simulink model "SMC"  (R2020b)
settings: Solver=VariableStepAuto  StartTime=0.0  StopTime=100  RelTol=1e-3
settings Model: Creator=Lenovo  LastModifiedBy=Lenovo
settings DataIOCC: ReturnWorkspaceOutputs=off
settings DebuggingCC: ArithmeticOperatorsInVariantConditions=warning
settings SFSimCC: SimUseLocalCustomCode=off  CustomCodeUndefinedFunction=UseInterfaceOnly
settings RTWCC: RTWUseLocalCustomCode=off

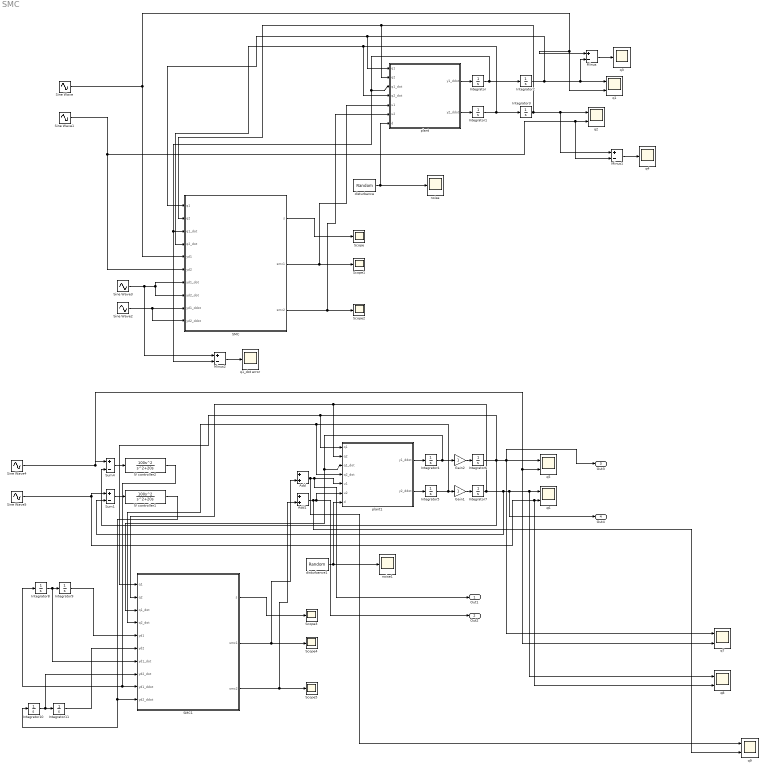
== system SMC ==
  Add : Sum
  Add1 : Sum
  Gain1 : Gain
  Gain2 : Gain
  IV controller1 : TransferFcn  Numerator=[100 0 0]  Denominator=[1 20 0]
  IV controller2 : TransferFcn  Numerator=[100 0 0]  Denominator=[1 20 0]
  Integrator{,1..11} (12 alike) : Integrator
  Minus : Sum  Inputs=+-
  Minus1 : Sum  Inputs=+-
  Minus2 : Sum  Inputs=+-
  SMC : MATLAB Function  TreatAsAtomicUnit=on
  SMC1 : MATLAB Function  TreatAsAtomicUnit=on
  Scope{,1..5} (6 alike) : Scope
  Sine Wave : Sin  Frequency=6  SampleTime=0.001
  Sine Wave1 : Sin  Frequency=6  SampleTime=0.001
  Sine Wave2 : Sin  Amplitude=-36  Frequency=6  SampleTime=0.001
  Sine Wave3 : Sin  Amplitude=6  Frequency=6  Phase=1.57  SampleTime=0.001
  Sine Wave4 : Sin  SampleTime=0.001
  Sine Wave5 : Sin  SampleTime=0.001
  Sum1 : Sum  Inputs=|+-
  Sum4 : Sum  Inputs=|+-
  disturbance : UniformRandomNumber  Minimum=0  Maximum=10  SampleTime=0.01
  disturbance1 : UniformRandomNumber  Minimum=-10  Maximum=10  SampleTime=0.001
  noise : Scope
  noise1 : Scope
  plant : MATLAB Function  TreatAsAtomicUnit=on
  plant1 : MATLAB Function  TreatAsAtomicUnit=on
  q{1..2,5..9} (7 alike) : Scope  NumInputPorts=2
  q1_dot error : Scope
  q3 : Scope
  q4 : Scope
  Out1 : Outport  VectorParamsAs1DForOutWhenUnconnected=off
  Out2 : Outport  Port=2  VectorParamsAs1DForOutWhenUnconnected=off
  Out3 : Outport  Port=3  VectorParamsAs1DForOutWhenUnconnected=off
  Out4 : Outport  Port=4  VectorParamsAs1DForOutWhenUnconnected=off
  wires:
  disturbance/1 -> plant/7(d), noise/1
  plant/2(y2_ddot) -> Integrator1/1
  SMC/1(s) -> Scope/1
  SMC/3(smc2) -> plant/6(u2), Scope2/1
  SMC/2(smc1) -> plant/5(u1), Scope1/1
  Integrator1/1 -> Integrator3/1, SMC/4(q2_dot), plant/4(q2_dot)
  plant/1(y1_ddot) -> Integrator/1
  Integrator2/1 -> Minus/2, q1/1, SMC/1(q1), plant/1(q1)
  Sine Wave/1 -> SMC/5(yd1), Minus/1, q1/2
  Sine Wave2/1 -> SMC/10(yd2_ddot), SMC/9(yd1_ddot)
  Minus/1 -> q3/1
  Sine Wave1/1 -> Minus1/2, q2/2, SMC/6(yd2)
  Integrator3/1 -> Minus1/1, q2/1, SMC/2(q2), plant/2(q2)
  Minus1/1 -> q4/1
  Integrator/1 -> Integrator2/1, Minus2/2, SMC/3(q1_dot), plant/3(q1_dot)
  Sine Wave3/1 -> Minus2/1, SMC/8(yd2_dot), SMC/7(yd1_dot)
  Minus2/1 -> q1_dot error/1
  Integrator11/1 -> SMC1/6(yd2)
  Sum1/1 -> IV controller1/1
  disturbance1/1 -> plant1/7(d), noise1/1
  Sine Wave5/1 -> q8/2, q6/2, Sum1/1
  Add1/1 -> q9/2, Out2/1, plant1/6(u2)
  Add/1 -> q9/1, Out1/1, plant1/5(u1)
  Integrator9/1 -> SMC1/5(yd1)
  SMC1/3(smc2) -> Add1/2, Scope5/1
  Integrator8/1 -> SMC1/7(yd1_dot), Integrator9/1
  Gain2/1 -> Integrator6/1
  Sine Wave4/1 -> q7/2, q5/2, Sum4/1
  IV controller2/1 -> Integrator8/1, SMC1/9(yd1_ddot)
  SMC1/1(s) -> Scope3/1
  IV controller1/1 -> Integrator10/1, SMC1/10(yd2_ddot)
  Sum4/1 -> IV controller2/1
  Integrator7/1 -> Out4/1, q8/1, q6/1, Sum1/2, SMC1/2(q2), plant1/2(q2)
  Integrator5/1 -> SMC1/4(q2_dot), plant1/4(q2_dot), Gain1/1
  plant1/1(y1_ddot) -> Integrator4/1
  Integrator4/1 -> Gain2/1, SMC1/3(q1_dot), plant1/3(q1_dot)
  Integrator10/1 -> SMC1/8(yd2_dot), Integrator11/1
  Integrator6/1 -> q7/1, Out3/1, q5/1, SMC1/1(q1), plant1/1(q1), Sum4/2
  Gain1/1 -> Integrator7/1
  SMC1/2(smc1) -> Add/2, Scope4/1
  plant1/2(y2_ddot) -> Integrator5/1

== matlab function SMC/SMC1 ==
  data: q1 input; s output; q2 input; q1_dot input; q2_dot input; smc1 output; yd1 input; yd2 input; yd1_dot input; yd2_dot input; yd1_ddot input; yd2_ddot input; smc2 output
function [s,smc1,smc2] = fcn(q1, q2, q1_dot, q2_dot, yd1,yd2,yd1_dot,yd2_dot,yd1_ddot,yd2_ddot)

m1 = 1; m2 = 1;
l1 = 1; l2 = 1;
g = 9.8;
c2 = cos(q2);
s2 = sin(q2);
h = -0.5*m2*l1*l2*s2;
c1 = cos(q1);
c2 = cos(q2);
c12 = cos(q1+q2);


H = [1/3*m1*l1*l1+m2*l1*l1+1/3*m2*l2*l2+m2*l1*l2*c2, 1/3*m2*l2*l2+0.5*m2*l1*l2*c2;
    1/3*m2*l2*l2+1/2*m2*l1*l2*c2, 1/3*m2*l2*l2];

C = [h*q2_dot, h*(q1_dot+q2_dot);
     -h*q1_dot, 0];
 
G = [0.5*m1*g*l1*c1+m2*g*l1*c1+0.5*m2*g*l2*c12;
     0.5*m2*g*l2*c12];

 
%%% smc
c1 = 10; c2 = 10; eita = 20;


z1 = [q1-yd1;q2-yd2];
z1_dot = [q1_dot-yd1_dot;q2_dot-yd2_dot];
z2 = c1 .* z1 + z1_dot;

%%%% sliding variable
s = z2;
sgn = s ./ (abs(s)+0.01);

%%%% control output
output = C * [q1_dot;q2_dot] + G + H * (-eita.*sgn-c1.*z1_dot+[yd1_ddot;yd2_ddot]-c2.*z2-z1);

smc1 = output(1,1);
smc2 = output(2,1);

== matlab function SMC/SMC ==
  data: q1 input; s output; q2 input; q1_dot input; q2_dot input; smc1 output; yd1 input; yd2 input; yd1_dot input; yd2_dot input; yd1_ddot input; yd2_ddot input; smc2 output
function [s,smc1,smc2] = fcn(q1, q2, q1_dot, q2_dot, yd1,yd2,yd1_dot,yd2_dot,yd1_ddot,yd2_ddot)

m1 = 1; m2 = 2;
l1 = 2; l2 = 2;
g = 9.8;
c2 = cos(q2);
s2 = sin(q2);
h = -0.5*m2*l1*l2*s2;
c1 = cos(q1);
c2 = cos(q2);
c12 = cos(q1+q2);


H = [1/3*m1*l1*l1+m2*l1*l1+1/3*m2*l2*l2+m2*l1*l2*c2, 1/3*m2*l2*l2+0.5*m2*l1*l2*c2;
    1/3*m2*l2*l2+1/2*m2*l1*l2*c2, 1/3*m2*l2*l2];

C = [h*q2_dot, h*(q1_dot+q2_dot);
     -h*q1_dot, 0];
 
G = [0.5*m1*g*l1*c1+m2*g*l1*c1+0.5*m2*g*l2*c12;
     0.5*m2*g*l2*c12];

 
%%% smc
c1 = 10; c2 = 10; eita = 20;


z1 = [q1-yd1;q2-yd2];
z1_dot = [q1_dot-yd1_dot;q2_dot-yd2_dot];
z2 = c1 .* z1 + z1_dot;

%%%% sliding variable
s = z2;
sgn = s ./ (abs(s)+0.01);

%%%% control output
output = C * [q1_dot;q2_dot] + G + H * (-eita.*sgn-c1.*z1_dot+[yd1_ddot;yd2_ddot]-c2.*z2-z1);

smc1 = output(1,1);
smc2 = output(2,1);

== matlab function SMC/plant ==
  data: q1 input; y1_ddot output; q2 input; q1_dot input; q2_dot input; y2_ddot output; u1 input; u2 input; d input
function [y1_ddot, y2_ddot] = fcn(q1, q2, q1_dot, q2_dot, u1, u2, d)

m1 = 1; m2 = 2;
l1 = 2; l2 = 2;
g = 9.8;
c2 = cos(q2);
s2 = sin(q2);
h = -0.5*m2*l1*l2*s2;
c1 = cos(q1);
c2 = cos(q2);
c12 = cos(q1+q2);


H = [1/3*m1*l1*l1+m2*l1*l1+1/3*m2*l2*l2+m2*l1*l2*c2, 1/3*m2*l2*l2+0.5*m2*l1*l2*c2;
    1/3*m2*l2*l2+1/2*m2*l1*l2*c2, 1/3*m2*l2*l2];

C = [h*q2_dot, h*(q1_dot+q2_dot);
     -h*q1_dot, 0];
 
G = [0.5*m1*g*l1*c1+m2*g*l1*c1+0.5*m2*g*l2*c12;
     0.5*m2*g*l2*c12];

output = inv(H) * ( [u1;u2] - C * [q1_dot;q2_dot] - G);

%%%%%% d means disturbance
y1_ddot = output(1,1) + d;
y2_ddot = output(2,1) + d;

== matlab function SMC/plant1 ==
  data: q1 input; y1_ddot output; q2 input; q1_dot input; q2_dot input; y2_ddot output; u1 input; u2 input; d input
function [y1_ddot, y2_ddot] = fcn(q1, q2, q1_dot, q2_dot, u1, u2, d)

m1 = 1; m2 = 1;
l1 = 1; l2 = 1;
g = 9.8;
c2 = cos(q2);
s2 = sin(q2);
h = -0.5*m2*l1*l2*s2;
c1 = cos(q1);
c2 = cos(q2);
c12 = cos(q1+q2);


H = [1/3*m1*l1*l1+m2*l1*l1+1/3*m2*l2*l2+m2*l1*l2*c2, 1/3*m2*l2*l2+0.5*m2*l1*l2*c2;
    1/3*m2*l2*l2+1/2*m2*l1*l2*c2, 1/3*m2*l2*l2];

C = [h*q2_dot, h*(q1_dot+q2_dot);
     -h*q1_dot, 0];
 
G = [0.5*m1*g*l1*c1+m2*g*l1*c1+0.5*m2*g*l2*c12;
     0.5*m2*g*l2*c12];

output = inv(H) * ( [u1;u2] - C * [q1_dot;q2_dot] - G);

%%%%%% d means disturbance
y1_ddot = output(1,1) + d;
y2_ddot = output(2,1) + d;
